simulink model "zadana"  (R2016a)
settings: Solver=ode4  StartTime=0.0  StopTime=30  FixedStep=0.001  RelTol=1e-3
settings Model: Creator=Student  LastModifiedBy=Maciek
settings DataIOCC: LimitDataPoints=on  SaveFormat=Array
settings HardwareCC: ProdBitPerPointer=32  ProdLargestAtomicFloat=None  ProdIntDivRoundTo=Undefined  ProdEndianess=Unspecified  ProdWordSize=32  ProdHWDeviceType=32-bit Generic
settings ModelReferenceCC: PropagateSignalLabelsOutOfModel=off
settings ConfigComp: CovModelRefEnable=Off

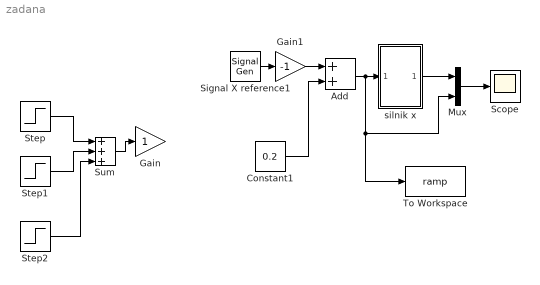
== system zadana ==
  Add : Sum
  Constant1 : Constant  Value=0.2
  Gain : Gain
  Gain1 : Gain  Gain=-1
  Mux : Mux  Inputs=2
  Scope : Scope
  Signal X reference1 : SignalGenerator  WaveForm=sawtooth  Amplitude=0.2  Frequency=0.02
  Step : Step  After=0.5  SampleTime=0
  Step1 : Step  Time=3  After=-0.5  SampleTime=0
  Step2 : Step  Time=6  After=-0.5  SampleTime=0
  Sum : Sum  Inputs=+++
  To Workspace : ToWorkspace  VariableName=ramp  SaveFormat=Timeseries  SampleTime=-1
  silnik x : Subsystem
  wires:
  Step/1 -> Sum/1
  Step1/1 -> Sum/2
  Step2/1 -> Sum/3
  Sum/1 -> Gain/1
  Constant1/1 -> Add/2
  Signal X reference1/1 -> Gain1/1
  Gain1/1 -> Add/1
  Add/1 -> To Workspace/1, Mux/2, silnik x/1(In1)
  silnik x/1(Out1) -> Mux/1
  Mux/1 -> Scope/1

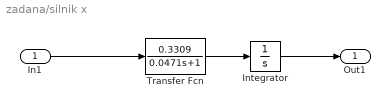
== system zadana/silnik x ==
  In1 : Inport
  Integrator : Integrator
  Transfer Fcn : TransferFcn  Numerator=0.3309  Denominator=[0.0471 1]
  Out1 : Outport
  wires:
  In1/1 -> Transfer Fcn/1
  Transfer Fcn/1 -> Integrator/1
  Integrator/1 -> Out1/1
